simulink model "lab5_q2_blockdiagram"  (Simulink 8.7)
settings: Solver=FixedStepDiscrete  StartTime=0.0  StopTime=40  RelTol=1e-3
values from neighbouring files (symbols this model uses):
  entrada = [0 1 1]    [lab5_q2_243886_262667.m]
  ys1 = [4 0 4]    [lab5_q2_243886_262667.m]
  ys2 = [0 0 0]    [lab5_q2_243886_262667.m]
settings Model: Creator=gmcma  LastModifiedBy=gmcma
settings DataIOCC: LimitDataPoints=off  SaveFormat=Dataset
settings DebuggingCC: UnderspecifiedInitializationDetection=Simplified  MergeDetectMultiDrivingBlocksExec=error
settings HardwareCC: ProdBitPerPointer=64  ProdLargestAtomicFloat=Float  ProdIntDivRoundTo=Zero  ProdEndianess=LittleEndian  ProdWordSize=64  ProdHWDeviceType=Intel->x86-64 (Windows64)
settings ModelReferenceCC: PropagateSignalLabelsOutOfModel=on
settings ConfigComp: CovModelRefEnable=off

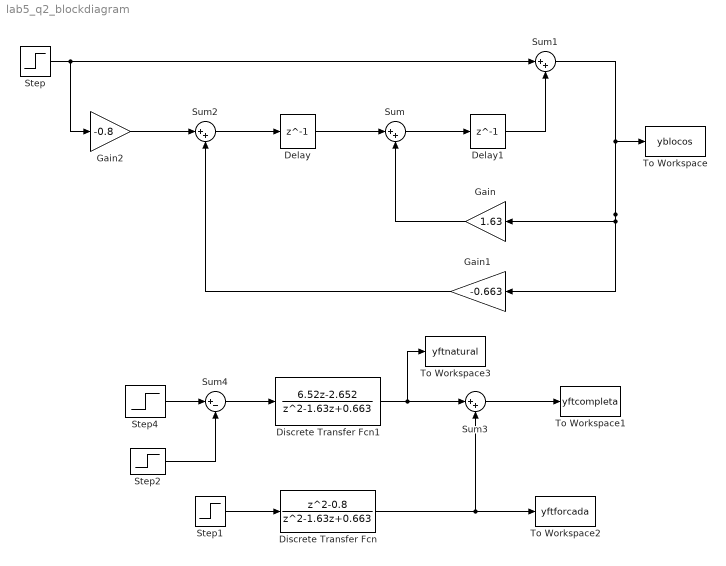
== system lab5_q2_blockdiagram ==
  Delay : Delay  DelayLength=1  InitialCondition=ys2
  Delay1 : Delay  DelayLength=1  InitialCondition=ys1
  Discrete Transfer Fcn : DiscreteTransferFcn  Numerator=[1 0 -0.8]  Denominator=[1 -1.63 0.663]  SampleTime=1
  Discrete Transfer Fcn1 : DiscreteTransferFcn  Numerator=[6.52 -2.652]  Denominator=[1 -1.63 0.663]  SampleTime=1
  Gain : Gain  Gain=1.63
  Gain1 : Gain  Gain=-0.663
  Gain2 : Gain  Gain=-0.8
  Step : Step  Time=0  After=entrada  SampleTime=1
  Step1 : Step  Time=0  SampleTime=1
  Step2 : Step  Time=0.001  SampleTime=0
  Step4 : Step  Time=0  SampleTime=0
  Sum{,1..3} (4 alike) : Sum  Inputs=|++
  Sum4 : Sum  Inputs=|+-
  To Workspace : ToWorkspace  VariableName=yblocos  SaveFormat=Structure With Time  SampleTime=-1
  To Workspace1 : ToWorkspace  VariableName=yftcompleta  SaveFormat=Structure With Time  SampleTime=-1
  To Workspace2 : ToWorkspace  VariableName=yftforcada  SaveFormat=Structure With Time  SampleTime=-1
  To Workspace3 : ToWorkspace  VariableName=yftnatural  SaveFormat=Structure With Time  SampleTime=1
  wires:
  Delay/1 -> Sum/1
  Sum/1 -> Delay1/1
  Delay1/1 -> Sum1/2
  Gain/1 -> Sum/2
  Sum2/1 -> Delay/1
  Gain1/1 -> Sum2/2
  Sum1/1 -> To Workspace/1, Gain1/1, Gain/1
  Gain2/1 -> Sum2/1
  Step/1 -> Gain2/1, Sum1/1
  Discrete Transfer Fcn/1 -> To Workspace2/1, Sum3/2
  Step1/1 -> Discrete Transfer Fcn/1
  Sum3/1 -> To Workspace1/1
  Discrete Transfer Fcn1/1 -> To Workspace3/1, Sum3/1
  Sum4/1 -> Discrete Transfer Fcn1/1
  Step4/1 -> Sum4/1
  Step2/1 -> Sum4/2
